simulink model "lag_sim"  (R2017b)
settings: Solver=ode45  StartTime=0.0  StopTime=10.0  RelTol=1e-3  EnableMultiTasking=on
undefined symbols (not defined in the file): K, K0
libraries: cstblocks x7, simulink x1
settings Model: Creator=ChrisJobling  LastModifiedBy=eechris
settings DataIOCC: LimitDataPoints=on  SaveFormat=Array
settings OptimizationCC: ExpressionDepthLimit=2147483647  LifeSpan=inf
settings DebuggingCC: UnderspecifiedInitializationDetection=Classic  MergeDetectMultiDrivingBlocksExec=none  SolverPrmCheckMsg=warning  StateNameClashWarn=warning  SFUnexpectedBacktrackingDiag=warning  SFNoUnconditionalDefaultTransitionDiag=warning  SFExecutionAtInitializationDiag=none
settings HardwareCC: ProdBitPerPointer=32  ProdBitPerSizeT=32  ProdBitPerPtrDiffT=32  ProdLargestAtomicFloat=None  ProdIntDivRoundTo=Undefined  ProdEndianess=Unspecified  ProdWordSize=32  ProdHWDeviceType=32-bit Generic
settings ModelReferenceCC: PropagateSignalLabelsOutOfModel=off
settings CodeAppCC: StateflowObjectComments=on
settings GRTTargetCC: TargetLangStandard=C89/C90 (ANSI)  GeneratePreprocessorConditionals=Disable all
settings ConfigComp: CovMetricSettings=dw  CovHtmlReporting=on  CovSaveCumulativeToWorkspaceVar=on  CovSaveSingleToWorkspaceVar=on  CovExternalEMLEnable=off

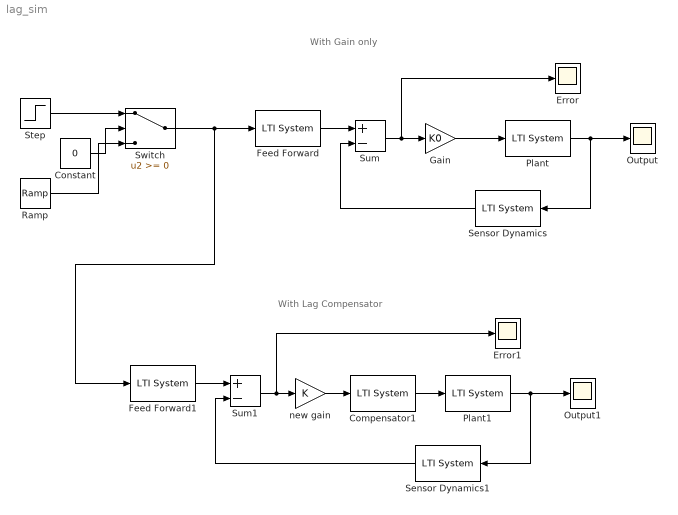
== system lag_sim ==
  note: With Gain only
  note: With Lag Compensator
  Compensator1 : cstblocks/LTI System  sys=Clag  IC=[]
  Constant : Constant  Value=0
  Error : Scope
  Error1 : Scope
  Feed Forward : cstblocks/LTI System  sys=F  IC=[]
  Feed Forward1 : cstblocks/LTI System  sys=F  IC=[]
  Gain : Gain  Gain=K0
  Output : Scope
  Output1 : Scope
  Plant : cstblocks/LTI System  sys=G  IC=[]
  Plant1 : cstblocks/LTI System  sys=G  IC=[]
  Ramp : simulink/Sources/Ramp  slope=1  start=0  X0=0
  Sensor Dynamics : cstblocks/LTI System  sys=H  IC=[]
  Sensor Dynamics1 : cstblocks/LTI System  sys=H  IC=[]
  Step : Step  Time=0  SampleTime=0
  Sum : Sum  Inputs=+-  SaturateOnIntegerOverflow=on  InputSameDT=on  OutDataTypeStr=Inherit: Same as first input
  Sum1 : Sum  Inputs=+-  SaturateOnIntegerOverflow=on  InputSameDT=on  OutDataTypeStr=Inherit: Same as first input
  Switch : Switch
  new gain : Gain  Gain=K
  wires:
  Feed Forward/1 -> Sum/1
  Sensor Dynamics/1 -> Sum/2
  Sum/1 -> Error/1, Gain/1
  Plant/1 -> Output/1, Sensor Dynamics/1
  Step/1 -> Switch/1
  Ramp/1 -> Switch/3
  Constant/1 -> Switch/2
  Feed Forward1/1 -> Sum1/1
  Sensor Dynamics1/1 -> Sum1/2
  Compensator1/1 -> Plant1/1
  Plant1/1 -> Sensor Dynamics1/1, Output1/1
  Gain/1 -> Plant/1
  Sum1/1 -> Error1/1, new gain/1
  new gain/1 -> Compensator1/1
  Switch/1 -> Feed Forward/1, Feed Forward1/1
